simulink model "problem_9"  (R2020b)
settings: Solver=VariableStepAuto  StartTime=0.0  StopTime=10.0  RelTol=1e-3
PreLoadFcn:
  | vars
values from neighbouring files (symbols this model uses):
  ke = 0.022    [vars.m]
  kf = 0.0002024    [vars.m]
  L = 0.001    [vars.m]
  R = 0.16    [vars.m]
undefined symbols (not defined in the file or in its folder): J
settings Model: Creator=hp  LastModifiedBy=hp

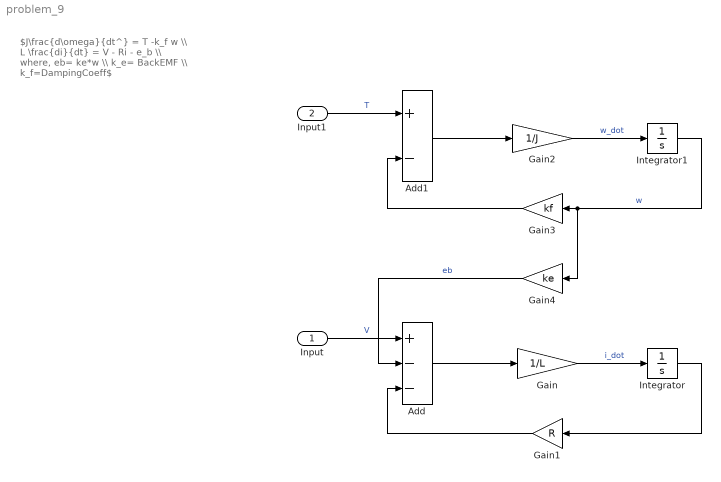
== system problem_9 ==
  note: $J\frac{d\omega}{dt^} = T -k_f w \\ L \frac{di}{dt} = V - Ri - e_b \\ where, eb= ke*w \\ k_e= BackEMF \\ k_f=DampingCoeff$
  Input : Inport
  Input1 : Inport  Port=2
  Add : Sum  Inputs=+--
  Add1 : Sum  Inputs=+-
  Gain : Gain  Gain=1/L
  Gain1 : Gain  Gain=R
  Gain2 : Gain  Gain=1/J
  Gain3 : Gain  Gain=kf
  Gain4 : Gain  Gain=ke
  Integrator : Integrator
  Integrator1 : Integrator
  wires:
  Add/1 -> Gain/1
  Gain/1 -> Integrator/1  "i_dot"
  Integrator/1 -> Gain1/1
  Gain1/1 -> Add/3
  Input/1 -> Add/1  "V"
  Add1/1 -> Gain2/1
  Gain2/1 -> Integrator1/1  "w_dot"
  Integrator1/1 -> Gain4/1, Gain3/1  "w"
  Gain3/1 -> Add1/2
  Input1/1 -> Add1/1  "T"
  Gain4/1 -> Add/2  "eb"
